simulink model "mod_firmware_NVH_v6"  (R2022a)
settings: Solver=FixedStepDiscrete  StartTime=0.0  StopTime=Inf  RelTol=1e-3  EnableMultiTasking=on
InitFcn:
  | params_NVH;
undefined symbols (not defined in the file): denz, DiscIntNeverNeededParam, Down, GPTRIP1SEL, GPTRIP2SEL, KiTs, Kp, numz, POS, rate_lim, target, Tper, Tref, Ts, TZ1, TZ2, Up
libraries: simulink x10, hdlsllib x7, mcbcontrolslib x5, c2802xlib x4, c2837xDlib x4, c280xlib x2, c2000lib x1, slpidlib x1
(part 2 of 2)

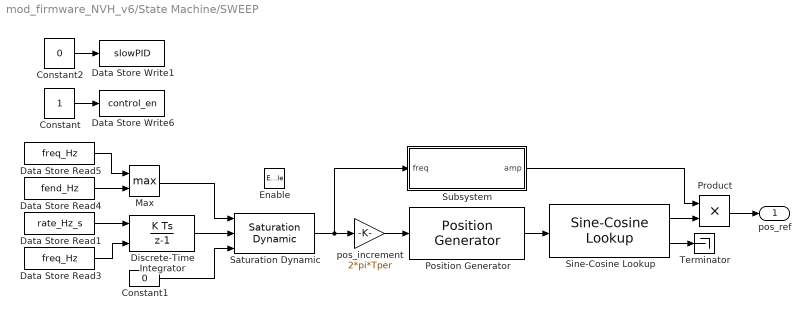
== system mod_firmware_NVH_v6/State Machine/SWEEP ==
  Enable : EnablePort  StatesWhenEnabling=reset
  Constant : Constant  OutDataTypeStr=boolean  SampleTime=Tper
  Constant1 : Constant  Value=0  OutDataTypeStr=single  SampleTime=Tper
  Constant2 : Constant  Value=0  OutDataTypeStr=boolean  SampleTime=Tper
  Data Store Read1 : DataStoreRead  DataStoreName=rate_Hz_s  SampleTime=Tper  IndexOptions=Index vector (dialog)  Indices=1  OutputSizes=1
  Data Store Read3 : DataStoreRead  DataStoreName=freq_Hz  SampleTime=Tper  IndexOptions=Index vector (dialog)  Indices=1  OutputSizes=1
  Data Store Read4 : DataStoreRead  DataStoreName=fend_Hz  SampleTime=Tper  IndexOptions=Index vector (dialog)  Indices=1  OutputSizes=1
  Data Store Read5 : DataStoreRead  DataStoreName=freq_Hz  SampleTime=Tper  IndexOptions=Index vector (dialog)  Indices=1  OutputSizes=1
  Data Store Write1 : DataStoreWrite  DataStoreName=slowPID  IndexOptions=Index vector (dialog)  Indices=1  OutputSizes=1
  Data Store Write6 : DataStoreWrite  DataStoreName=control_en  IndexOptions=Index vector (dialog)  Indices=1  OutputSizes=1
  Discrete-Time Integrator : DiscreteIntegrator  InitialConditionSource=external  InitialCondition=4  SampleTime=-1  LimitOutput=on  UpperSaturationLimit=100  LowerSaturationLimit=0  ICPrevOutput=DiscIntNeverNeededParam  ICPrevScaledInput=DiscIntNeverNeededParam
  Max : MinMax  Function=max  Inputs=2
  Position Generator : mcbcontrolslib/Position Generator  AngleOutput=Radians  ThetaSource=External  ThetaInput=5e-4  DataType=double  ExternalReset=none  Offset=0
      settings: SourceProductBaseCode=MT
  Product : Product
  Saturation Dynamic : simulink/Discontinuities/Saturation Dynamic  OutMin=[]  OutMax=[]  OutDataTypeStr=Inherit: Same as second input  OutDataType=fixdt(1, 16)  OutScaling=2^-10  DoSatur=off
  Sine-Cosine Lookup : mcbcontrolslib/Sine-Cosine Lookup  AngleInput=Radians  N_points=1024
      settings: SourceProductBaseCode=MT
  Subsystem : Subsystem
  Terminator : Terminator
  pos_increment : Gain  Gain=2*pi*Tper  RndMeth=Simplest  OutDataTypeStr=Inherit: Same as input
  pos_ref : Outport
  wires:
  Sine-Cosine Lookup/2 -> Terminator/1
  Position Generator/1 -> Sine-Cosine Lookup/1
  Saturation Dynamic/1 -> Subsystem/1(freq), pos_increment/1
  Sine-Cosine Lookup/1 -> Product/2
  pos_increment/1 -> Position Generator/1
  Constant/1 -> Data Store Write6/1
  Data Store Read1/1 -> Discrete-Time Integrator/1
  Product/1 -> pos_ref/1
  Constant2/1 -> Data Store Write1/1
  Data Store Read3/1 -> Discrete-Time Integrator/2
  Discrete-Time Integrator/1 -> Saturation Dynamic/2
  Constant1/1 -> Saturation Dynamic/3
  Data Store Read4/1 -> Max/2
  Data Store Read5/1 -> Max/1
  Max/1 -> Saturation Dynamic/1
  Subsystem/1(amp) -> Product/1

== system mod_firmware_NVH_v6/Current Control/ADC sampling/Convert ==
  ADC : Inport
  Constant : Constant  Value=POS.offset  OutDataTypeStr=single
  Data Type Conversion1 : DataTypeConversion  OutDataTypeStr=dataType  ConvertRealWorld=Stored Integer (SI)  RndMeth=Simplest  SaturateOnIntegerOverflow=off
  Gain : Gain  Gain=POS.gain  OutDataTypeStr=dataType  RndMeth=Simplest
  Sum : Sum  Inputs=|+-
  mm : Outport
  wires:
  ADC/1 -> Data Type Conversion1/1
  Constant/1 -> Sum/2
  Data Type Conversion1/1 -> Gain/1
  Gain/1 -> Sum/1
  Sum/1 -> mm/1

== system mod_firmware_NVH_v6/Current Control/Data Serial Output/Data ==
  Data : Inport
  Data_width : Inport  Port=2
  Action Port : ActionPort  ActionPortLabel=else
  Mux : Mux  Inputs=2
  Start : Constant  Value=hex2dec('0000')  OutDataTypeStr=uint16
  Data_out : Outport  VectorParamsAs1DForOutWhenUnconnected=off
  Iteration : Outport  Port=2  VectorParamsAs1DForOutWhenUnconnected=off
  wires:
  Start/1 -> Mux/2
  Mux/1 -> Data_out/1
  Data/1 -> Mux/1
  Data_width/1 -> Iteration/1

== system mod_firmware_NVH_v6/Current Control/Data Serial Output/End ==
  Data : Inport
  Data_width : Inport  Port=2
  Action Port : ActionPort  ActionPortLabel=elseif(u1 == 999)
  Bias : Bias  Bias=1  SaturateOnIntegerOverflow=off
  Mux : Mux  Inputs=2
  Start : Constant  Value=hex2dec('4545')  OutDataTypeStr=uint16
  Data_out : Outport  VectorParamsAs1DForOutWhenUnconnected=off
  Iteration : Outport  Port=2  VectorParamsAs1DForOutWhenUnconnected=off
  wires:
  Mux/1 -> Data_out/1
  Data_width/1 -> Bias/1
  Start/1 -> Mux/2
  Bias/1 -> Iteration/1
  Data/1 -> Mux/1

== system mod_firmware_NVH_v6/Current Control/Data Serial Output/Start ==
  Data : Inport
  Data_width : Inport  Port=2
  Action Port : ActionPort  ActionPortLabel=if(u1 == 0)
  Bias : Bias  Bias=1  SaturateOnIntegerOverflow=off
  End : Constant  Value=hex2dec('5353')  OutDataTypeStr=uint16
  Mux : Mux  Inputs=2
  Data_out : Outport  VectorParamsAs1DForOutWhenUnconnected=off
  Iteration : Outport  Port=2  VectorParamsAs1DForOutWhenUnconnected=off
  wires:
  End/1 -> Mux/1
  Mux/1 -> Data_out/1
  Data_width/1 -> Bias/1
  Bias/1 -> Iteration/1
  Data/1 -> Mux/2

== system mod_firmware_NVH_v6/Current Control/Data Serial Output/While Iterator Subsystem ==
  Data : Inport
  Iteration : Inport  Port=2
  Add : Sum  Inputs=+-  OutDataTypeStr=Inherit: Same as first input
  Index Vector : MultiPortSwitch  Inputs=1  SaturateOnIntegerOverflow=off  InputSameDT=off
  SCI Transmit : c280xlib/SCI Transmit  sciModule=A  dataHead=''  dataTail=''  blockingMode=on  outputStatus=off
  While Iterator : WhileIterator  MaxIters=-1  WhileBlockType=do-while  ShowIterationPort=on  OutputDataType=int16
  wires:
  Iteration/1 -> Add/1
  Add/1 -> While Iterator/1
  Index Vector/1 -> SCI Transmit/1
  Data/1 -> Index Vector/2
  While Iterator/1 -> Index Vector/1, Add/2

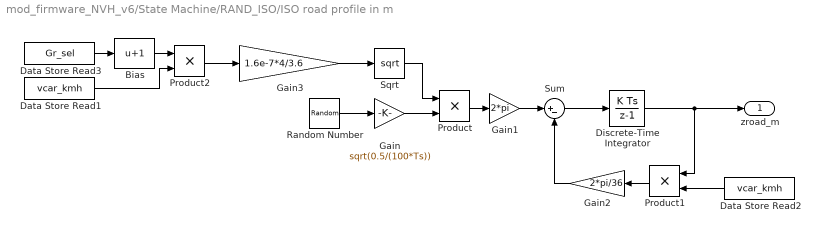
== system mod_firmware_NVH_v6/State Machine/RAND_ISO/ISO road profile in m ==
  Bias : Bias  Bias=1  SaturateOnIntegerOverflow=off
  Data Store Read1 : DataStoreRead  DataStoreName=vcar_kmh  SampleTime=Tref  IndexOptions=Index vector (dialog)  Indices=1  OutputSizes=1
  Data Store Read2 : DataStoreRead  DataStoreName=vcar_kmh  SampleTime=Tref  IndexOptions=Index vector (dialog)  Indices=1  OutputSizes=1
  Data Store Read3 : DataStoreRead  DataStoreName=Gr_sel  SampleTime=Tref  IndexOptions=Index vector (dialog)  Indices=1  OutputSizes=1
  Discrete-Time Integrator : DiscreteIntegrator  SampleTime=-1  ICPrevOutput=DiscIntNeverNeededParam  ICPrevScaledInput=DiscIntNeverNeededParam
  Gain : Gain  Gain=sqrt(0.5/(100*Ts))  OutDataTypeStr=single
  Gain1 : Gain  Gain=2*pi  OutDataTypeStr=single
  Gain2 : Gain  Gain=2*pi/36  OutDataTypeStr=single
  Gain3 : Gain  Gain=1.6e-7*4/3.6
  Product : Product
  Product1 : Product
  Product2 : Product
  Random Number : RandomNumber  Seed=23341  SampleTime=Tref
  Sqrt : Sqrt
  Sum : Sum  Inputs=|+-
  zroad_m : Outport
  wires:
  Random Number/1 -> Gain/1
  Product/1 -> Gain1/1
  Data Store Read2/1 -> Product1/2
  Gain3/1 -> Sqrt/1
  Gain1/1 -> Sum/1
  Gain2/1 -> Sum/2
  Gain/1 -> Product/2
  Data Store Read1/1 -> Product2/2
  Product2/1 -> Gain3/1
  Sum/1 -> Discrete-Time Integrator/1
  Discrete-Time Integrator/1 -> zroad_m/1, Product1/1
  Product1/1 -> Gain2/1
  Sqrt/1 -> Product/1
  Bias/1 -> Product2/1
  Data Store Read3/1 -> Bias/1

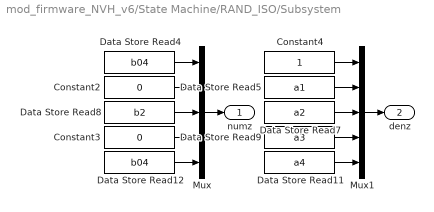
== system mod_firmware_NVH_v6/State Machine/RAND_ISO/Subsystem ==
  Constant2 : Constant  Value=0  OutDataTypeStr=single  SampleTime=Tref
  Constant3 : Constant  Value=0  OutDataTypeStr=single  SampleTime=Tref
  Constant4 : Constant  OutDataTypeStr=single  SampleTime=Tref
  Data Store Read11 : DataStoreRead  DataStoreName=a4  SampleTime=Tref  IndexOptions=Index vector (dialog)  Indices=1  OutputSizes=1
  Data Store Read12 : DataStoreRead  DataStoreName=b04  SampleTime=Tref  IndexOptions=Index vector (dialog)  Indices=1  OutputSizes=1
  Data Store Read4 : DataStoreRead  DataStoreName=b04  SampleTime=Tref  IndexOptions=Index vector (dialog)  Indices=1  OutputSizes=1
  Data Store Read5 : DataStoreRead  DataStoreName=a1  SampleTime=Tref  IndexOptions=Index vector (dialog)  Indices=1  OutputSizes=1
  Data Store Read7 : DataStoreRead  DataStoreName=a2  SampleTime=Tref  IndexOptions=Index vector (dialog)  Indices=1  OutputSizes=1
  Data Store Read8 : DataStoreRead  DataStoreName=b2  SampleTime=Tref  IndexOptions=Index vector (dialog)  Indices=1  OutputSizes=1
  Data Store Read9 : DataStoreRead  DataStoreName=a3  SampleTime=Tref  IndexOptions=Index vector (dialog)  Indices=1  OutputSizes=1
  Mux : Mux  Inputs=5
  Mux1 : Mux  Inputs=5
  numz : Outport
  denz : Outport  Port=2
  wires:
  Data Store Read8/1 -> Mux/3
  Data Store Read11/1 -> Mux1/5
  Data Store Read7/1 -> Mux1/3
  Data Store Read9/1 -> Mux1/4
  Data Store Read5/1 -> Mux1/2
  Constant3/1 -> Mux/4
  Constant2/1 -> Mux/2
  Constant4/1 -> Mux1/1
  Data Store Read12/1 -> Mux/5
  Data Store Read4/1 -> Mux/1
  Mux1/1 -> denz/1
  Mux/1 -> numz/1

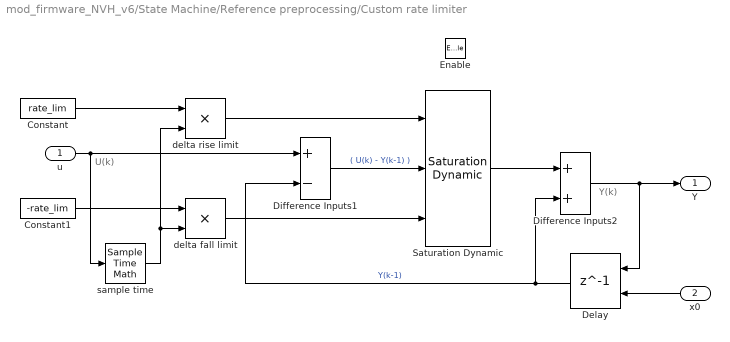
== system mod_firmware_NVH_v6/State Machine/Reference preprocessing/Custom rate limiter ==
  note: Y(k)
  note: U(k)
  u : Inport
  x0 : Inport  Port=2
  Enable : EnablePort  StatesWhenEnabling=reset
  Constant : Constant  Value=rate_lim
  Constant1 : Constant  Value=-rate_lim
  Delay : Delay  DelayLength=1  InitialConditionSource=Input port
      settings: InputPortMap=u0,p4
  Difference Inputs1 : Sum  Description=Add in CPU  DisableCoverage=on  Inputs=+-  OutDataTypeStr=Inherit: Inherit via back propagation
  Difference Inputs2 : Sum  Description=Add in CPU  OutDataTypeStr=Inherit: Inherit via back propagation
  Saturation Dynamic : simulink/Discontinuities/Saturation Dynamic  OutMin=[]  OutMax=[]  OutDataTypeStr=Inherit: Same as second input  OutDataType=fixdt(1, 16)  OutScaling=2^-10  DoSatur=off
  delta fall limit : Product  DisableCoverage=on  Inputs=**  OutDataTypeStr=Inherit: Inherit via back propagation  SaturateOnIntegerOverflow=on
  delta rise limit : Product  DisableCoverage=on  Inputs=**  OutDataTypeStr=Inherit: Inherit via back propagation  SaturateOnIntegerOverflow=on
  sample time : SampleTimeMath  DisableCoverage=on  TsampMathOp=Ts Only  weightValue=1
  Y : Outport  InitialOutput=0
  wires:
  Constant/1 -> delta rise limit/1
  Difference Inputs2/1 -> Delay/1, Y/1
  delta rise limit/1 -> Saturation Dynamic/1
  u/1 -> Difference Inputs1/1, sample time/1
  Difference Inputs1/1 -> Saturation Dynamic/2  "( U(k) - Y(k-1) )"
  x0/1 -> Delay/2
  Delay/1 -> Difference Inputs1/2, Difference Inputs2/2  "Y(k-1)"
  sample time/1 -> delta fall limit/2, delta rise limit/2
  Constant1/1 -> delta fall limit/1
  Saturation Dynamic/1 -> Difference Inputs2/1
  delta fall limit/1 -> Saturation Dynamic/3

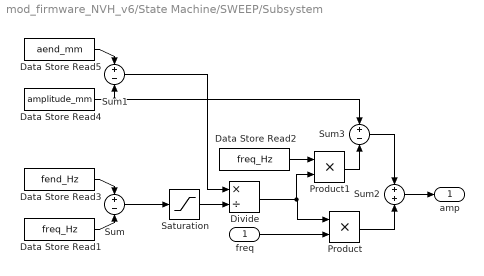
== system mod_firmware_NVH_v6/State Machine/SWEEP/Subsystem ==
  freq : Inport
  Data Store Read1 : DataStoreRead  DataStoreName=freq_Hz  SampleTime=Tper  IndexOptions=Index vector (dialog)  Indices=1  OutputSizes=1
  Data Store Read2 : DataStoreRead  DataStoreName=freq_Hz  SampleTime=Tper  IndexOptions=Index vector (dialog)  Indices=1  OutputSizes=1
  Data Store Read3 : DataStoreRead  DataStoreName=fend_Hz  SampleTime=Tper  IndexOptions=Index vector (dialog)  Indices=1  OutputSizes=1
  Data Store Read4 : DataStoreRead  DataStoreName=amplitude_mm  SampleTime=Tper  IndexOptions=Index vector (dialog)  Indices=1  OutputSizes=1
  Data Store Read5 : DataStoreRead  DataStoreName=aend_mm  SampleTime=Tper  IndexOptions=Index vector (dialog)  Indices=1  OutputSizes=1
  Divide : Product  Inputs=*/
  Product : Product
  Product1 : Product
  Saturation : Saturate  UpperLimit=inf  LowerLimit=0.1
  Sum : Sum  Inputs=+-
  Sum1 : Sum  Inputs=+-
  Sum2 : Sum
  Sum3 : Sum  Inputs=+-
  amp : Outport
  wires:
  Sum2/1 -> amp/1
  Data Store Read3/1 -> Sum/1
  Data Store Read1/1 -> Sum/2
  Sum/1 -> Saturation/1
  Saturation/1 -> Divide/2
  Sum1/1 -> Divide/1
  Data Store Read5/1 -> Sum1/1
  Data Store Read4/1 -> Sum3/1, Sum1/2
  Divide/1 -> Product1/2, Product/1
  freq/1 -> Product/2
  Product/1 -> Sum2/2
  Sum3/1 -> Sum2/1
  Data Store Read2/1 -> Product1/1
  Product1/1 -> Sum3/2

== stateflow chart mod_firmware_NVH_v6/State Machine/Chart ==
  state POWER_OFF
    during:
    state = -1;
  state POWER_ON
    during:
    state = 0;
  state POSITIONING
    during:
    state = 1;
  state SINE
    during:
    state = 2;
  state ERROR
    during:
    state = -2;
  state SWEEP
    during:
    state = 3;
  state RAND_ISO
    during:
    state = 4;
  state PROFILE
    during:
    state = 5;
  ERROR -> POWER_OFF : [fault == 0]
  POWER_OFF -> ERROR [order 1] : [fault == 1]
  SINE -> POWER_OFF [order 2] : [pow_en == 0]
  POSITIONING -> ERROR [order 3] : [fault == 1]
  POSITIONING -> POWER_OFF [order 6] : [pow_en == 0]
  SINE -> ERROR [order 1] : [fault == 1]
  (default) -> POWER_OFF
  POWER_ON -> POWER_OFF [order 2] : [pow_en == 0]
  POWER_ON -> POSITIONING [order 1] : [pos_en == 1]
  POSITIONING -> SINE [order 1] : [test_sel == 0 && test_start == 1]
  SINE -> POSITIONING [order 3] : [test_stop == 1]
  POWER_OFF -> POWER_ON [order 2] : [pow_en==1]
  PROFILE -> ERROR [order 1] : [fault == 1]
  RAND_ISO -> ERROR [order 1] : [fault == 1]
  SWEEP -> ERROR [order 2] : [fault == 1]
  SWEEP -> POSITIONING [order 1] : [test_stop == 1]
  PROFILE -> POWER_OFF [order 2] : [pow_en == 0]
  RAND_ISO -> POWER_OFF [order 2] : [pow_en == 0]
  SWEEP -> POWER_OFF [order 3] : [pow_en == 0]
  POSITIONING -> PROFILE [order 4] : [test_sel == 3 && test_start == 1]
  PROFILE -> POSITIONING [order 3] : [test_stop == 1]
  POSITIONING -> RAND_ISO [order 5] : [test_sel == 2 && test_start == 1]
  RAND_ISO -> POSITIONING [order 3] : [test_stop == 1]
  POSITIONING -> SWEEP [order 2] : [test_sel == 1 && test_start == 1]
  data: fault input; pow_en input; pos_en input; test_sel input; test_start input; test_stop input; state output single
